simulink model "psocintegralcontrol"  (R2024b)
settings: Solver=VariableStepAuto  StartTime=0.0  StopTime=10.0  RelTol=1e-3
libraries: spspowerguiLib x1
settings Model: Creator=ASUS  LastModifiedBy=ASUS

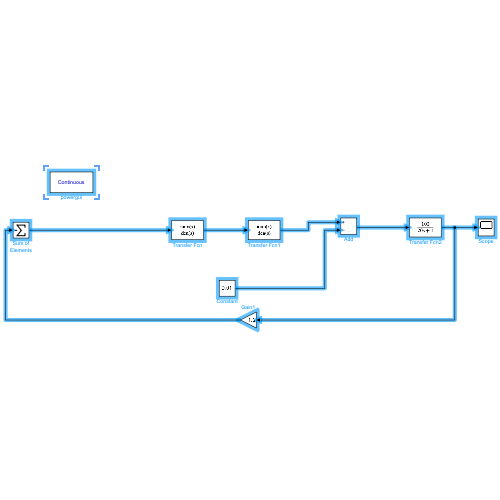
[thumbnail: Simulink's stored preview of the top-level diagram]
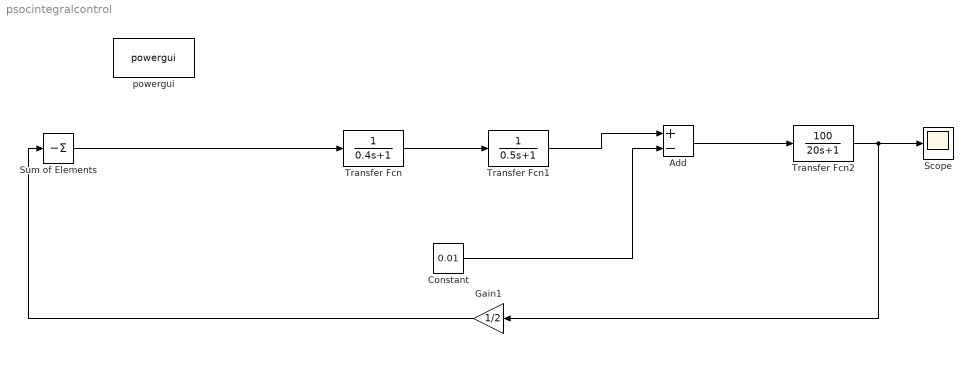
== system psocintegralcontrol ==
  Add : Sum  Inputs=+-
  Constant : Constant  Value=0.01
  Gain1 : Gain  Gain=1/2
  Scope : Scope
  Sum of Elements : Sum  Inputs=-
  Transfer Fcn : TransferFcn  Denominator=[0.4 1]  ParameterTunability=Optimized
  Transfer Fcn1 : TransferFcn  Denominator=[0.5 1]  ParameterTunability=Optimized
  Transfer Fcn2 : TransferFcn  Numerator=[100]  Denominator=[20 1]
  powergui : spspowerguiLib/powergui  Priority=1  SimulationMode=Continuous  SampleTime=50e-6  frequency=60  Iterations=50  frequencyindice=60  Pbase=100e6  ErrMax=1e-4  UnitsV=kV  UnitsW=MW  buscounter=0  FunctionMessages=off  echomessages=off  EnableUseOfTLC=off  CurrentSourceSwitches=off  DisableSnubberDevices=off  DisableRonSwitches=off  DisableVfSwitches=off  DisplayEquations=off  AutomaticDiscreteSolvers=off  SolverType=Tustin/Backward Euler (TBE)  Interpol=off  ExternalGateDelay=off  methode=off  Ts=100  x0status=blocks  SPID=on  SwTol=0  HookPort=off  NonlinearTolerance=1e-4  nMaxIteration=100  ContinueOnMaxIteration=off  RestoreLinks=warning  ResistiveCurrentMeasurement=off  Frange=[0:2:500]  Ylog=off  Xlog=on  ShowGrid=off  save=off  variable=ZData  structure=0  ZoomFFT=off  StartTime=0.0  cycles=1  DisplayStyle=1  fundamental=60  FreqAxis=off  MaxFrequency=1000  frequencyindicesteady=1  RmsSteady=1  display=off
  wires:
  Transfer Fcn/1 -> Transfer Fcn1/1
  Transfer Fcn1/1 -> Add/1
  Constant/1 -> Add/2
  Add/1 -> Transfer Fcn2/1
  Transfer Fcn2/1 -> Gain1/1, Scope/1
  Sum of Elements/1 -> Transfer Fcn/1
  Gain1/1 -> Sum of Elements/1
